simulink library "xps_library"  (R2012b)
settings: Solver=ode45  SolverMode=SingleTasking  StartTime=0.0  StopTime=10.0  RelTol=1e-3
undefined symbols (not defined in the file): sys_clk, xps_library_software_register_user_data_in
libraries: xbsIndex_r4 x788, simulink x100, dspsigops x81, casper_library x62, xps_library x24, casper_library_misc x3, xbsIndex_r3 x2
(part 5 of 9)

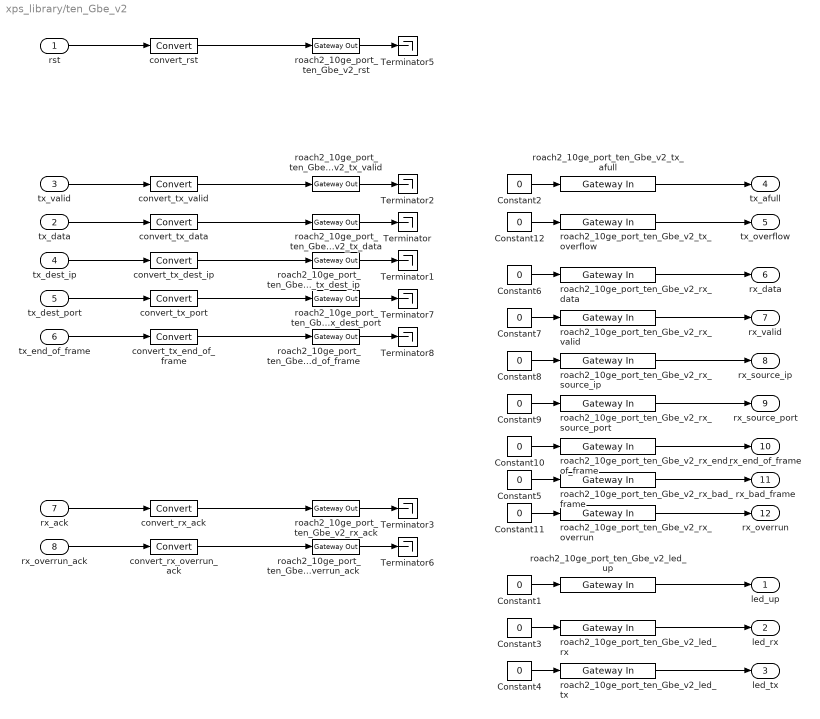
== system xps_library/ten_Gbe_v2 ==
  rst : Inport
  tx_data : Inport  Port=2
  tx_valid : Inport  Port=3
  tx_dest_ip : Inport  Port=4
  tx_dest_port : Inport  Port=5
  tx_end_of_frame : Inport  Port=6
  rx_ack : Inport  Port=7
  rx_overrun_ack : Inport  Port=8
  Constant{1..12} (12 alike) : Constant  Value=0
  Terminator{,1..3,5..8} (8 alike) : Terminator
  convert_rst : xbsIndex_r4/Convert  arith_type=Boolean  n_bits=64  bin_pt=0  quantization=Truncate  overflow=Wrap  latency=0  dbl_ovrd=off  pipeline=off  block_type=convert
      settings: xl_area=[0, 0, 0, 0, 0, 0, 0]
  convert_rx_ack : xbsIndex_r4/Convert  arith_type=Boolean  n_bits=64  bin_pt=0  quantization=Truncate  overflow=Wrap  latency=0  dbl_ovrd=off  pipeline=off  block_type=convert
      settings: xl_area=[0, 0, 0, 0, 0, 0, 0]
  convert_rx_overrun_ack : xbsIndex_r4/Convert  arith_type=Boolean  n_bits=64  bin_pt=0  quantization=Truncate  overflow=Wrap  latency=0  dbl_ovrd=off  pipeline=off  block_type=convert
      settings: xl_area=[0, 0, 0, 0, 0, 0, 0]
  convert_tx_data : xbsIndex_r4/Convert  arith_type=Unsigned  n_bits=64  bin_pt=0  quantization=Truncate  overflow=Wrap  latency=0  dbl_ovrd=off  pipeline=off  block_type=convert
      settings: xl_area=[0, 0, 0, 0, 0, 0, 0]
  convert_tx_dest_ip : xbsIndex_r4/Convert  arith_type=Unsigned  n_bits=32  bin_pt=0  quantization=Truncate  overflow=Wrap  latency=0  dbl_ovrd=off  pipeline=off  block_type=convert
      settings: xl_area=[0, 0, 0, 0, 0, 0, 0]
  convert_tx_end_of_frame : xbsIndex_r4/Convert  arith_type=Boolean  n_bits=1  bin_pt=0  quantization=Truncate  overflow=Wrap  latency=0  dbl_ovrd=off  pipeline=off  block_type=convert
      settings: xl_area=[0, 0, 0, 0, 0, 0, 0]
  convert_tx_port : xbsIndex_r4/Convert  arith_type=Unsigned  n_bits=16  bin_pt=0  quantization=Truncate  overflow=Wrap  latency=0  dbl_ovrd=off  pipeline=off  block_type=convert
      settings: xl_area=[0, 0, 0, 0, 0, 0, 0]
  convert_tx_valid : xbsIndex_r4/Convert  arith_type=Boolean  n_bits=1  bin_pt=0  quantization=Truncate  overflow=Wrap  latency=0  dbl_ovrd=off  pipeline=off  block_type=convert
      settings: xl_area=[0, 0, 0, 0, 0, 0, 0]
  roach2_10ge_port_ten_Gbe_v2_led_rx : xbsIndex_r4/Gateway In  arith_type=Boolean  n_bits=1  bin_pt=0  quantization=Truncate  overflow=Wrap  period=1  dbl_ovrd=off  timing_constraint=None  locs_specified=off  LOCs={}  hdl_port=on  block_type=gatewayin
      settings: infoedit="Gateway in block.  Converts inputs of type Simulink integer, double and fixed point to  Xilinx fixed point type.<P><P>Hardware notes:  In hardware these blocks become top level input ports."  xl_area=[0, 0, 0, 0, 0, 0, 0]
  roach2_10ge_port_ten_Gbe_v2_led_tx : xbsIndex_r4/Gateway In  arith_type=Boolean  n_bits=1  bin_pt=0  quantization=Truncate  overflow=Wrap  period=1  dbl_ovrd=off  timing_constraint=None  locs_specified=off  LOCs={}  hdl_port=on  block_type=gatewayin
      settings: infoedit="Gateway in block.  Converts inputs of type Simulink integer, double and fixed point to  Xilinx fixed point type.<P><P>Hardware notes:  In hardware these blocks become top level input ports."  xl_area=[0, 0, 0, 0, 0, 0, 0]
  roach2_10ge_port_ten_Gbe_v2_led_up : xbsIndex_r4/Gateway In  arith_type=Boolean  n_bits=1  bin_pt=0  quantization=Truncate  overflow=Wrap  period=1  dbl_ovrd=off  timing_constraint=None  locs_specified=off  LOCs={}  hdl_port=on  block_type=gatewayin
      settings: infoedit="Gateway in block.  Converts inputs of type Simulink integer, double and fixed point to  Xilinx fixed point type.<P><P>Hardware notes:  In hardware these blocks become top level input ports."  xl_area=[0, 0, 0, 0, 0, 0, 0]
  roach2_10ge_port_ten_Gbe_v2_rst : xbsIndex_r4/Gateway Out  hdl_port=on  timing_constraint=None  locs_specified=off  LOCs={}  block_type=gatewayout
      settings: infoedit="Gateway out block.  Converts Xilinx fixed point inputs into ouputs of type Simulink integer, double, or fixed point.<P><P>Hardware notes:  In hardware these blocks become top level output ports or are discarded, depending on how they are configured."  xl_area=[0, 0, 0, 0, 0, 0, 0]
  roach2_10ge_port_ten_Gbe_v2_rx_ack : xbsIndex_r4/Gateway Out  hdl_port=on  timing_constraint=None  locs_specified=off  LOCs={}  block_type=gatewayout
      settings: infoedit="Gateway out block.  Converts Xilinx fixed point inputs into ouputs of type Simulink integer, double, or fixed point.<P><P>Hardware notes:  In hardware these blocks become top level output ports or are discarded, depending on how they are configured."  xl_area=[0, 0, 0, 0, 0, 0, 0]
  roach2_10ge_port_ten_Gbe_v2_rx_bad_frame : xbsIndex_r4/Gateway In  arith_type=Boolean  n_bits=1  bin_pt=0  quantization=Truncate  overflow=Wrap  period=1  dbl_ovrd=off  timing_constraint=None  locs_specified=off  LOCs={}  hdl_port=on  block_type=gatewayin
      settings: infoedit="Gateway in block.  Converts inputs of type Simulink integer, double and fixed point to  Xilinx fixed point type.<P><P>Hardware notes:  In hardware these blocks become top level input ports."  xl_area=[0, 0, 0, 0, 0, 0, 0]
  roach2_10ge_port_ten_Gbe_v2_rx_data : xbsIndex_r4/Gateway In  arith_type=Unsigned  n_bits=64  bin_pt=0  quantization=Truncate  overflow=Wrap  period=1  dbl_ovrd=off  timing_constraint=None  locs_specified=off  LOCs={}  hdl_port=on  block_type=gatewayin
      settings: infoedit="Gateway in block.  Converts inputs of type Simulink integer, double and fixed point to  Xilinx fixed point type.<P><P>Hardware notes:  In hardware these blocks become top level input ports."  xl_area=[0, 0, 0, 0, 0, 0, 0]
  roach2_10ge_port_ten_Gbe_v2_rx_end_of_frame : xbsIndex_r4/Gateway In  arith_type=Boolean  n_bits=1  bin_pt=0  quantization=Truncate  overflow=Wrap  period=1  dbl_ovrd=off  timing_constraint=None  locs_specified=off  LOCs={}  hdl_port=on  block_type=gatewayin
      settings: infoedit="Gateway in block.  Converts inputs of type Simulink integer, double and fixed point to  Xilinx fixed point type.<P><P>Hardware notes:  In hardware these blocks become top level input ports."  xl_area=[0, 0, 0, 0, 0, 0, 0]
  roach2_10ge_port_ten_Gbe_v2_rx_overrun : xbsIndex_r4/Gateway In  arith_type=Boolean  n_bits=1  bin_pt=0  quantization=Truncate  overflow=Wrap  period=1  dbl_ovrd=off  timing_constraint=None  locs_specified=off  LOCs={}  hdl_port=on  block_type=gatewayin
      settings: infoedit="Gateway in block.  Converts inputs of type Simulink integer, double and fixed point to  Xilinx fixed point type.<P><P>Hardware notes:  In hardware these blocks become top level input ports."  xl_area=[0, 0, 0, 0, 0, 0, 0]
  roach2_10ge_port_ten_Gbe_v2_rx_overrun_ack : xbsIndex_r4/Gateway Out  hdl_port=on  timing_constraint=None  locs_specified=off  LOCs={}  block_type=gatewayout
      settings: infoedit="Gateway out block.  Converts Xilinx fixed point inputs into ouputs of type Simulink integer, double, or fixed point.<P><P>Hardware notes:  In hardware these blocks become top level output ports or are discarded, depending on how they are configured."  xl_area=[0, 0, 0, 0, 0, 0, 0]
  roach2_10ge_port_ten_Gbe_v2_rx_source_ip : xbsIndex_r4/Gateway In  arith_type=Unsigned  n_bits=32  bin_pt=0  quantization=Truncate  overflow=Wrap  period=1  dbl_ovrd=off  timing_constraint=None  locs_specified=off  LOCs={}  hdl_port=on  block_type=gatewayin
      settings: infoedit="Gateway in block.  Converts inputs of type Simulink integer, double and fixed point to  Xilinx fixed point type.<P><P>Hardware notes:  In hardware these blocks become top level input ports."  xl_area=[0, 0, 0, 0, 0, 0, 0]
  roach2_10ge_port_ten_Gbe_v2_rx_source_port : xbsIndex_r4/Gateway In  arith_type=Unsigned  n_bits=16  bin_pt=0  quantization=Truncate  overflow=Wrap  period=1  dbl_ovrd=off  timing_constraint=None  locs_specified=off  LOCs={}  hdl_port=on  block_type=gatewayin
      settings: infoedit="Gateway in block.  Converts inputs of type Simulink integer, double and fixed point to  Xilinx fixed point type.<P><P>Hardware notes:  In hardware these blocks become top level input ports."  xl_area=[0, 0, 0, 0, 0, 0, 0]
  roach2_10ge_port_ten_Gbe_v2_rx_valid : xbsIndex_r4/Gateway In  arith_type=Boolean  n_bits=1  bin_pt=0  quantization=Truncate  overflow=Wrap  period=1  dbl_ovrd=off  timing_constraint=None  locs_specified=off  LOCs={}  hdl_port=on  block_type=gatewayin
      settings: infoedit="Gateway in block.  Converts inputs of type Simulink integer, double and fixed point to  Xilinx fixed point type.<P><P>Hardware notes:  In hardware these blocks become top level input ports."  xl_area=[0, 0, 0, 0, 0, 0, 0]
  roach2_10ge_port_ten_Gbe_v2_tx_afull : xbsIndex_r4/Gateway In  arith_type=Boolean  n_bits=1  bin_pt=0  quantization=Truncate  overflow=Wrap  period=1  dbl_ovrd=off  timing_constraint=None  locs_specified=off  LOCs={}  hdl_port=on  block_type=gatewayin
      settings: infoedit="Gateway in block.  Converts inputs of type Simulink integer, double and fixed point to  Xilinx fixed point type.<P><P>Hardware notes:  In hardware these blocks become top level input ports."  xl_area=[0, 0, 0, 0, 0, 0, 0]
  roach2_10ge_port_ten_Gbe_v2_tx_data : xbsIndex_r4/Gateway Out  hdl_port=on  timing_constraint=None  locs_specified=off  LOCs={}  block_type=gatewayout
      settings: infoedit="Gateway out block.  Converts Xilinx fixed point inputs into ouputs of type Simulink integer, double, or fixed point.<P><P>Hardware notes:  In hardware these blocks become top level output ports or are discarded, depending on how they are configured."  xl_area=[0, 0, 0, 0, 0, 0, 0]
  roach2_10ge_port_ten_Gbe_v2_tx_dest_ip : xbsIndex_r4/Gateway Out  hdl_port=on  timing_constraint=None  locs_specified=off  LOCs={}  block_type=gatewayout
      settings: infoedit="Gateway out block.  Converts Xilinx fixed point inputs into ouputs of type Simulink integer, double, or fixed point.<P><P>Hardware notes:  In hardware these blocks become top level output ports or are discarded, depending on how they are configured."  xl_area=[0, 0, 0, 0, 0, 0, 0]
  roach2_10ge_port_ten_Gbe_v2_tx_dest_port : xbsIndex_r4/Gateway Out  hdl_port=on  timing_constraint=None  locs_specified=off  LOCs={}  block_type=gatewayout
      settings: infoedit="Gateway out block.  Converts Xilinx fixed point inputs into ouputs of type Simulink integer, double, or fixed point.<P><P>Hardware notes:  In hardware these blocks become top level output ports or are discarded, depending on how they are configured."  xl_area=[0, 0, 0, 0, 0, 0, 0]
  roach2_10ge_port_ten_Gbe_v2_tx_end_of_frame : xbsIndex_r4/Gateway Out  hdl_port=on  timing_constraint=None  locs_specified=off  LOCs={}  block_type=gatewayout
      settings: infoedit="Gateway out block.  Converts Xilinx fixed point inputs into ouputs of type Simulink integer, double, or fixed point.<P><P>Hardware notes:  In hardware these blocks become top level output ports or are discarded, depending on how they are configured."  xl_area=[0, 0, 0, 0, 0, 0, 0]
  roach2_10ge_port_ten_Gbe_v2_tx_overflow : xbsIndex_r4/Gateway In  arith_type=Boolean  n_bits=1  bin_pt=0  quantization=Truncate  overflow=Wrap  period=1  dbl_ovrd=off  timing_constraint=None  locs_specified=off  LOCs={}  hdl_port=on  block_type=gatewayin
      settings: infoedit="Gateway in block.  Converts inputs of type Simulink integer, double and fixed point to  Xilinx fixed point type.<P><P>Hardware notes:  In hardware these blocks become top level input ports."  xl_area=[0, 0, 0, 0, 0, 0, 0]
  roach2_10ge_port_ten_Gbe_v2_tx_valid : xbsIndex_r4/Gateway Out  hdl_port=on  timing_constraint=None  locs_specified=off  LOCs={}  block_type=gatewayout
      settings: infoedit="Gateway out block.  Converts Xilinx fixed point inputs into ouputs of type Simulink integer, double, or fixed point.<P><P>Hardware notes:  In hardware these blocks become top level output ports or are discarded, depending on how they are configured."  xl_area=[0, 0, 0, 0, 0, 0, 0]
  led_up : Outport
  led_rx : Outport  Port=2
  led_tx : Outport  Port=3
  tx_afull : Outport  Port=4
  tx_overflow : Outport  Port=5
  rx_data : Outport  Port=6
  rx_valid : Outport  Port=7
  rx_source_ip : Outport  Port=8
  rx_source_port : Outport  Port=9
  rx_end_of_frame : Outport  Port=10
  rx_bad_frame : Outport  Port=11
  rx_overrun : Outport  Port=12
  wires:
  roach2_10ge_port_ten_Gbe_v2_led_tx/1 -> led_tx/1
  Constant4/1 -> roach2_10ge_port_ten_Gbe_v2_led_tx/1
  roach2_10ge_port_ten_Gbe_v2_led_rx/1 -> led_rx/1
  Constant3/1 -> roach2_10ge_port_ten_Gbe_v2_led_rx/1
  roach2_10ge_port_ten_Gbe_v2_led_up/1 -> led_up/1
  Constant1/1 -> roach2_10ge_port_ten_Gbe_v2_led_up/1
  roach2_10ge_port_ten_Gbe_v2_rx_end_of_frame/1 -> rx_end_of_frame/1
  Constant10/1 -> roach2_10ge_port_ten_Gbe_v2_rx_end_of_frame/1
  roach2_10ge_port_ten_Gbe_v2_rx_source_port/1 -> rx_source_port/1
  Constant9/1 -> roach2_10ge_port_ten_Gbe_v2_rx_source_port/1
  Constant8/1 -> roach2_10ge_port_ten_Gbe_v2_rx_source_ip/1
  roach2_10ge_port_ten_Gbe_v2_rx_source_ip/1 -> rx_source_ip/1
  roach2_10ge_port_ten_Gbe_v2_tx_end_of_frame/1 -> Terminator8/1
  convert_tx_end_of_frame/1 -> roach2_10ge_port_ten_Gbe_v2_tx_end_of_frame/1
  tx_end_of_frame/1 -> convert_tx_end_of_frame/1
  roach2_10ge_port_ten_Gbe_v2_tx_dest_port/1 -> Terminator7/1
  convert_tx_port/1 -> roach2_10ge_port_ten_Gbe_v2_tx_dest_port/1
  tx_dest_port/1 -> convert_tx_port/1
  roach2_10ge_port_ten_Gbe_v2_rst/1 -> Terminator5/1
  convert_rst/1 -> roach2_10ge_port_ten_Gbe_v2_rst/1
  rst/1 -> convert_rst/1
  roach2_10ge_port_ten_Gbe_v2_rx_valid/1 -> rx_valid/1
  Constant7/1 -> roach2_10ge_port_ten_Gbe_v2_rx_valid/1
  roach2_10ge_port_ten_Gbe_v2_rx_ack/1 -> Terminator3/1
  Constant6/1 -> roach2_10ge_port_ten_Gbe_v2_rx_data/1
  Constant2/1 -> roach2_10ge_port_ten_Gbe_v2_tx_afull/1
  roach2_10ge_port_ten_Gbe_v2_tx_valid/1 -> Terminator2/1
  roach2_10ge_port_ten_Gbe_v2_tx_dest_ip/1 -> Terminator1/1
  roach2_10ge_port_ten_Gbe_v2_tx_data/1 -> Terminator/1
  roach2_10ge_port_ten_Gbe_v2_tx_afull/1 -> tx_afull/1
  convert_tx_valid/1 -> roach2_10ge_port_ten_Gbe_v2_tx_valid/1
  tx_valid/1 -> convert_tx_valid/1
  convert_tx_dest_ip/1 -> roach2_10ge_port_ten_Gbe_v2_tx_dest_ip/1
  tx_dest_ip/1 -> convert_tx_dest_ip/1
  convert_tx_data/1 -> roach2_10ge_port_ten_Gbe_v2_tx_data/1
  tx_data/1 -> convert_tx_data/1
  roach2_10ge_port_ten_Gbe_v2_rx_data/1 -> rx_data/1
  convert_rx_ack/1 -> roach2_10ge_port_ten_Gbe_v2_rx_ack/1
  rx_ack/1 -> convert_rx_ack/1
  roach2_10ge_port_ten_Gbe_v2_rx_bad_frame/1 -> rx_bad_frame/1
  Constant5/1 -> roach2_10ge_port_ten_Gbe_v2_rx_bad_frame/1
  roach2_10ge_port_ten_Gbe_v2_rx_overrun/1 -> rx_overrun/1
  Constant11/1 -> roach2_10ge_port_ten_Gbe_v2_rx_overrun/1
  roach2_10ge_port_ten_Gbe_v2_rx_overrun_ack/1 -> Terminator6/1
  convert_rx_overrun_ack/1 -> roach2_10ge_port_ten_Gbe_v2_rx_overrun_ack/1
  rx_overrun_ack/1 -> convert_rx_overrun_ack/1
  Constant12/1 -> roach2_10ge_port_ten_Gbe_v2_tx_overflow/1
  roach2_10ge_port_ten_Gbe_v2_tx_overflow/1 -> tx_overflow/1

== system xps_library/ADCs/adc083000_ctrl ==
  conf : Inport
  sdata_bus : Inport  Port=2
  Convert : xbsIndex_r4/Convert  arith_type=Unsigned  n_bits=3  bin_pt=0  quantization=Truncate  overflow=Wrap  latency=2  dbl_ovrd=off  pipeline=off  block_type=convert
      settings: block_version=11.4
  Convert1 : xbsIndex_r4/Convert  arith_type=Unsigned  n_bits=32  bin_pt=0  quantization=Truncate  overflow=Wrap  latency=2  dbl_ovrd=off  pipeline=off  block_type=convert
      settings: block_version=11.4
  Slice : xbsIndex_r4/Slice  nbits=3  boolean_output=off  mode=Lower Bit Location + Width  bit1=0  base1=MSB of Input  bit0=0  base0=LSB of Input  dbl_ovrd=off  block_type=slice
  Terminator : Terminator
  Terminator1 : Terminator
  xps_library_ADCs_adc083000_ctrl_conf : xbsIndex_r4/Gateway Out  hdl_port=on  timing_constraint=None  locs_specified=off  LOCs={}  block_type=gatewayout
      settings: infoedit="Gateway out block.  Converts Xilinx fixed point inputs into ouputs of type Simulink integer, double, or fixed point.<br><br>Hardware notes:  In hardware these blocks become top level output ports or are discarded, depending on how they are configured."  block_version=11.4
  xps_library_ADCs_adc083000_ctrl_sdata_bus : xbsIndex_r4/Gateway Out  hdl_port=on  timing_constraint=None  locs_specified=off  LOCs={}  block_type=gatewayout
      settings: infoedit="Gateway out block.  Converts Xilinx fixed point inputs into ouputs of type Simulink integer, double, or fixed point.<br><br>Hardware notes:  In hardware these blocks become top level output ports or are discarded, depending on how they are configured."  block_version=11.4
  wires:
  xps_library_ADCs_adc083000_ctrl_sdata_bus/1 -> Terminator1/1
  xps_library_ADCs_adc083000_ctrl_conf/1 -> Terminator/1
  Convert1/1 -> xps_library_ADCs_adc083000_ctrl_sdata_bus/1
  Slice/1 -> Convert/1
  conf/1 -> Slice/1
  Convert/1 -> xps_library_ADCs_adc083000_ctrl_conf/1
  sdata_bus/1 -> Convert1/1

== system xps_library/ADCs/adc2x14_400 ==
  adc_snap_test_zdock0_adc2x14_400_user_data_i0 : xbsIndex_r4/Gateway In  arith_type=Unsigned  n_bits=14  bin_pt=0  quantization=Truncate  overflow=Wrap  period=1  dbl_ovrd=off  timing_constraint=None  locs_specified=off  LOCs={}  hdl_port=on  block_type=gatewayin
      settings: infoedit="Gateway in block.  Converts inputs of type Simulink integer, double and fixed point to  Xilinx fixed point type.<P><P>Hardware notes:  In hardware these blocks become top level input ports."  xl_area=[0, 0, 0, 0, 0, 0, 0]  block_version=10.1.3
  adc_snap_test_zdock0_adc2x14_400_user_data_i1 : xbsIndex_r4/Gateway In  arith_type=Unsigned  n_bits=14  bin_pt=0  quantization=Truncate  overflow=Wrap  period=1  dbl_ovrd=off  timing_constraint=None  locs_specified=off  LOCs={}  hdl_port=on  block_type=gatewayin
      settings: infoedit="Gateway in block.  Converts inputs of type Simulink integer, double and fixed point to  Xilinx fixed point type.<P><P>Hardware notes:  In hardware these blocks become top level input ports."  xl_area=[0, 0, 0, 0, 0, 0, 0]  block_version=10.1.3
  adc_snap_test_zdock0_adc2x14_400_user_data_q0 : xbsIndex_r4/Gateway In  arith_type=Unsigned  n_bits=14  bin_pt=0  quantization=Truncate  overflow=Wrap  period=1  dbl_ovrd=off  timing_constraint=None  locs_specified=off  LOCs={}  hdl_port=on  block_type=gatewayin
      settings: infoedit="Gateway in block.  Converts inputs of type Simulink integer, double and fixed point to  Xilinx fixed point type.<P><P>Hardware notes:  In hardware these blocks become top level input ports."  xl_area=[0, 0, 0, 0, 0, 0, 0]  block_version=10.1.3
  adc_snap_test_zdock0_adc2x14_400_user_data_q1 : xbsIndex_r4/Gateway In  arith_type=Unsigned  n_bits=14  bin_pt=0  quantization=Truncate  overflow=Wrap  period=1  dbl_ovrd=off  timing_constraint=None  locs_specified=off  LOCs={}  hdl_port=on  block_type=gatewayin
      settings: infoedit="Gateway in block.  Converts inputs of type Simulink integer, double and fixed point to  Xilinx fixed point type.<P><P>Hardware notes:  In hardware these blocks become top level input ports."  xl_area=[0, 0, 0, 0, 0, 0, 0]  block_version=10.1.3
  adc_snap_test_zdock0_adc2x14_400_user_sync : xbsIndex_r4/Gateway In  arith_type=Boolean  n_bits=1  bin_pt=0  quantization=Truncate  overflow=Wrap  period=1  dbl_ovrd=off  timing_constraint=None  locs_specified=off  LOCs={}  hdl_port=on  block_type=gatewayin
      settings: infoedit="Gateway in block.  Converts inputs of type Simulink integer, double and fixed point to  Xilinx fixed point type.<P><P>Hardware notes:  In hardware these blocks become top level input ports."  xl_area=[0, 0, 0, 0, 0, 0, 0]  block_version=10.1.3
  conv : Subsystem
      mask help:
      | Converts an (12-bit) unsigned number to 2's complement.
      | This block should eventually be able to handle arbitrary
      | width inputs.
  conv1 : Subsystem
      mask help:
      | Converts an (12-bit) unsigned number to 2's complement.
      | This block should eventually be able to handle arbitrary
      | width inputs.
  conv2 : Subsystem
      mask help:
      | Converts an (12-bit) unsigned number to 2's complement.
      | This block should eventually be able to handle arbitrary
      | width inputs.
  conv3 : Subsystem
      mask help:
      | Converts an (12-bit) unsigned number to 2's complement.
      | This block should eventually be able to handle arbitrary
      | width inputs.
  data_i0 : Outport
  data_i1 : Outport  Port=2
  data_q0 : Outport  Port=3
  data_q1 : Outport  Port=4
  sync : Outport  Port=5
  wires:
  adc_snap_test_zdock0_adc2x14_400_user_sync/1 -> sync/1
  adc_snap_test_zdock0_adc2x14_400_user_data_i0/1 -> conv/1(In1)
  conv/1(Out1) -> data_i0/1
  adc_snap_test_zdock0_adc2x14_400_user_data_q0/1 -> conv2/1(In1)
  conv2/1(Out1) -> data_q0/1
  adc_snap_test_zdock0_adc2x14_400_user_data_i1/1 -> conv1/1(In1)
  conv1/1(Out1) -> data_i1/1
  adc_snap_test_zdock0_adc2x14_400_user_data_q1/1 -> conv3/1(In1)
  conv3/1(Out1) -> data_q1/1

== system xps_library/ADCs/adc2x14_400_4x ==
  conv : Subsystem
      mask help:
      | Converts an (14-bit) unsigned number to 2's complement.
      | This block should eventually be able to handle arbitrary
      | width inputs.
  conv1 : Subsystem
      mask help:
      | Converts an (14-bit) unsigned number to 2's complement.
      | This block should eventually be able to handle arbitrary
      | width inputs.
  conv2 : Subsystem
      mask help:
      | Converts an (14-bit) unsigned number to 2's complement.
      | This block should eventually be able to handle arbitrary
      | width inputs.
  conv3 : Subsystem
      mask help:
      | Converts an (14-bit) unsigned number to 2's complement.
      | This block should eventually be able to handle arbitrary
      | width inputs.
  conv4 : Subsystem
      mask help:
      | Converts an (14-bit) unsigned number to 2's complement.
      | This block should eventually be able to handle arbitrary
      | width inputs.
  conv5 : Subsystem
      mask help:
      | Converts an (14-bit) unsigned number to 2's complement.
      | This block should eventually be able to handle arbitrary
      | width inputs.
  conv6 : Subsystem
      mask help:
      | Converts an (14-bit) unsigned number to 2's complement.
      | This block should eventually be able to handle arbitrary
      | width inputs.
  conv7 : Subsystem
      mask help:
      | Converts an (14-bit) unsigned number to 2's complement.
      | This block should eventually be able to handle arbitrary
      | width inputs.
  xps_library_ADCs_adc2x14_400_4x_user_data_i{0..3} (4 alike) : xbsIndex_r4/Gateway In  arith_type=Unsigned  n_bits=14  bin_pt=0  quantization=Truncate  overflow=Wrap  period=1  dbl_ovrd=off  timing_constraint=None  locs_specified=off  LOCs={}  block_type=gatewayin
      settings: infoedit="Gateway in block.  Converts inputs of type Simulink integer, double and fixed point to  Xilinx fixed point type.<P><P>Hardware notes:  In hardware these blocks become top level input ports."  xl_area=[0, 0, 0, 0, 0, 0, 0]  block_version=10.1.3
  xps_library_ADCs_adc2x14_400_4x_user_data_q{0..3} (4 alike) : xbsIndex_r4/Gateway In  arith_type=Unsigned  n_bits=14  bin_pt=0  quantization=Truncate  overflow=Wrap  period=1  dbl_ovrd=off  timing_constraint=None  locs_specified=off  LOCs={}  block_type=gatewayin
      settings: infoedit="Gateway in block.  Converts inputs of type Simulink integer, double and fixed point to  Xilinx fixed point type.<P><P>Hardware notes:  In hardware these blocks become top level input ports."  xl_area=[0, 0, 0, 0, 0, 0, 0]  block_version=10.1.3
  xps_library_ADCs_adc2x14_400_4x_user_sync : xbsIndex_r4/Gateway In  arith_type=Boolean  n_bits=1  bin_pt=0  quantization=Truncate  overflow=Wrap  period=1  dbl_ovrd=off  timing_constraint=None  locs_specified=off  LOCs={}  block_type=gatewayin
      settings: infoedit="Gateway in block.  Converts inputs of type Simulink integer, double and fixed point to  Xilinx fixed point type.<P><P>Hardware notes:  In hardware these blocks become top level input ports."  xl_area=[0, 0, 0, 0, 0, 0, 0]  block_version=10.1.3
  data_i0 : Outport
  data_i1 : Outport  Port=2
  data_i2 : Outport  Port=3
  data_i3 : Outport  Port=4
  data_q0 : Outport  Port=5
  data_q1 : Outport  Port=6
  data_q2 : Outport  Port=7
  data_q3 : Outport  Port=8
  sync : Outport  Port=9
  wires:
  conv5/1(Out1) -> data_q1/1
  xps_library_ADCs_adc2x14_400_4x_user_data_q1/1 -> conv5/1(In1)
  conv1/1(Out1) -> data_i1/1
  xps_library_ADCs_adc2x14_400_4x_user_data_i1/1 -> conv1/1(In1)
  conv4/1(Out1) -> data_q0/1
  xps_library_ADCs_adc2x14_400_4x_user_data_q0/1 -> conv4/1(In1)
  conv/1(Out1) -> data_i0/1
  xps_library_ADCs_adc2x14_400_4x_user_data_i0/1 -> conv/1(In1)
  xps_library_ADCs_adc2x14_400_4x_user_sync/1 -> sync/1
  conv2/1(Out1) -> data_i2/1
  xps_library_ADCs_adc2x14_400_4x_user_data_i2/1 -> conv2/1(In1)
  conv3/1(Out1) -> data_i3/1
  xps_library_ADCs_adc2x14_400_4x_user_data_i3/1 -> conv3/1(In1)
  conv6/1(Out1) -> data_q2/1
  xps_library_ADCs_adc2x14_400_4x_user_data_q2/1 -> conv6/1(In1)
  conv7/1(Out1) -> data_q3/1
  xps_library_ADCs_adc2x14_400_4x_user_data_q3/1 -> conv7/1(In1)

== system xps_library/ADCs/adc_mkid ==
  conv : Subsystem
      mask help:
      | Converts an (12-bit) unsigned number to 2's complement.
      | This block should eventually be able to handle arbitrary
      | width inputs.
  conv1 : Subsystem
      mask help:
      | Converts an (12-bit) unsigned number to 2's complement.
      | This block should eventually be able to handle arbitrary
      | width inputs.
  conv2 : Subsystem
      mask help:
      | Converts an (12-bit) unsigned number to 2's complement.
      | This block should eventually be able to handle arbitrary
      | width inputs.
  conv3 : Subsystem
      mask help:
      | Converts an (12-bit) unsigned number to 2's complement.
      | This block should eventually be able to handle arbitrary
      | width inputs.
  xps_library_ADCs_adc_mkid_user_data_i0 : xbsIndex_r4/Gateway In  arith_type=Unsigned  n_bits=12  bin_pt=0  quantization=Truncate  overflow=Wrap  period=1  dbl_ovrd=off  timing_constraint=None  locs_specified=off  LOCs={}  hdl_port=on  block_type=gatewayin
      settings: infoedit="Gateway in block.  Converts inputs of type Simulink integer, double and fixed point to  Xilinx fixed point type.<P><P>Hardware notes:  In hardware these blocks become top level input ports."  xl_area=[0, 0, 0, 0, 0, 0, 0]  block_version=10.1.3
  xps_library_ADCs_adc_mkid_user_data_i1 : xbsIndex_r4/Gateway In  arith_type=Unsigned  n_bits=12  bin_pt=0  quantization=Truncate  overflow=Wrap  period=1  dbl_ovrd=off  timing_constraint=None  locs_specified=off  LOCs={}  hdl_port=on  block_type=gatewayin
      settings: infoedit="Gateway in block.  Converts inputs of type Simulink integer, double and fixed point to  Xilinx fixed point type.<P><P>Hardware notes:  In hardware these blocks become top level input ports."  xl_area=[0, 0, 0, 0, 0, 0, 0]  block_version=10.1.3
  xps_library_ADCs_adc_mkid_user_data_q0 : xbsIndex_r4/Gateway In  arith_type=Unsigned  n_bits=12  bin_pt=0  quantization=Truncate  overflow=Wrap  period=1  dbl_ovrd=off  timing_constraint=None  locs_specified=off  LOCs={}  hdl_port=on  block_type=gatewayin
      settings: infoedit="Gateway in block.  Converts inputs of type Simulink integer, double and fixed point to  Xilinx fixed point type.<P><P>Hardware notes:  In hardware these blocks become top level input ports."  xl_area=[0, 0, 0, 0, 0, 0, 0]  block_version=10.1.3
  xps_library_ADCs_adc_mkid_user_data_q1 : xbsIndex_r4/Gateway In  arith_type=Unsigned  n_bits=12  bin_pt=0  quantization=Truncate  overflow=Wrap  period=1  dbl_ovrd=off  timing_constraint=None  locs_specified=off  LOCs={}  hdl_port=on  block_type=gatewayin
      settings: infoedit="Gateway in block.  Converts inputs of type Simulink integer, double and fixed point to  Xilinx fixed point type.<P><P>Hardware notes:  In hardware these blocks become top level input ports."  xl_area=[0, 0, 0, 0, 0, 0, 0]  block_version=10.1.3
  xps_library_ADCs_adc_mkid_user_sync : xbsIndex_r4/Gateway In  arith_type=Boolean  n_bits=1  bin_pt=0  quantization=Truncate  overflow=Wrap  period=1  dbl_ovrd=off  timing_constraint=None  locs_specified=off  LOCs={}  hdl_port=on  block_type=gatewayin
      settings: infoedit="Gateway in block.  Converts inputs of type Simulink integer, double and fixed point to  Xilinx fixed point type.<P><P>Hardware notes:  In hardware these blocks become top level input ports."  xl_area=[0, 0, 0, 0, 0, 0, 0]  block_version=10.1.3
  data_i0 : Outport
  data_i1 : Outport  Port=2
  data_q0 : Outport  Port=3
  data_q1 : Outport  Port=4
  sync : Outport  Port=5
  wires:
  xps_library_ADCs_adc_mkid_user_sync/1 -> sync/1
  xps_library_ADCs_adc_mkid_user_data_i0/1 -> conv/1(In1)
  conv/1(Out1) -> data_i0/1
  xps_library_ADCs_adc_mkid_user_data_q0/1 -> conv2/1(In1)
  conv2/1(Out1) -> data_q0/1
  xps_library_ADCs_adc_mkid_user_data_i1/1 -> conv1/1(In1)
  conv1/1(Out1) -> data_i1/1
  xps_library_ADCs_adc_mkid_user_data_q1/1 -> conv3/1(In1)
  conv3/1(Out1) -> data_q1/1

== system xps_library/ADCs/adc_mkid_4x ==
  conv : Subsystem
      mask help:
      | Converts an (12-bit) unsigned number to 2's complement.
      | This block should eventually be able to handle arbitrary
      | width inputs.
  conv1 : Subsystem
      mask help:
      | Converts an (12-bit) unsigned number to 2's complement.
      | This block should eventually be able to handle arbitrary
      | width inputs.
  conv2 : Subsystem
      mask help:
      | Converts an (12-bit) unsigned number to 2's complement.
      | This block should eventually be able to handle arbitrary
      | width inputs.
  conv3 : Subsystem
      mask help:
      | Converts an (12-bit) unsigned number to 2's complement.
      | This block should eventually be able to handle arbitrary
      | width inputs.
  conv4 : Subsystem
      mask help:
      | Converts an (12-bit) unsigned number to 2's complement.
      | This block should eventually be able to handle arbitrary
      | width inputs.
  conv5 : Subsystem
      mask help:
      | Converts an (12-bit) unsigned number to 2's complement.
      | This block should eventually be able to handle arbitrary
      | width inputs.
  conv6 : Subsystem
      mask help:
      | Converts an (12-bit) unsigned number to 2's complement.
      | This block should eventually be able to handle arbitrary
      | width inputs.
  conv7 : Subsystem
      mask help:
      | Converts an (12-bit) unsigned number to 2's complement.
      | This block should eventually be able to handle arbitrary
      | width inputs.
  xps_library_ADCs_adc_mkid_4x_user_data_i{0..3} (4 alike) : xbsIndex_r4/Gateway In  arith_type=Unsigned  n_bits=12  bin_pt=0  quantization=Truncate  overflow=Wrap  period=1  dbl_ovrd=off  timing_constraint=None  locs_specified=off  LOCs={}  block_type=gatewayin
      settings: infoedit="Gateway in block.  Converts inputs of type Simulink integer, double and fixed point to  Xilinx fixed point type.<P><P>Hardware notes:  In hardware these blocks become top level input ports."  xl_area=[0, 0, 0, 0, 0, 0, 0]  block_version=10.1.3
  xps_library_ADCs_adc_mkid_4x_user_data_q{0..3} (4 alike) : xbsIndex_r4/Gateway In  arith_type=Unsigned  n_bits=12  bin_pt=0  quantization=Truncate  overflow=Wrap  period=1  dbl_ovrd=off  timing_constraint=None  locs_specified=off  LOCs={}  block_type=gatewayin
      settings: infoedit="Gateway in block.  Converts inputs of type Simulink integer, double and fixed point to  Xilinx fixed point type.<P><P>Hardware notes:  In hardware these blocks become top level input ports."  xl_area=[0, 0, 0, 0, 0, 0, 0]  block_version=10.1.3
  xps_library_ADCs_adc_mkid_4x_user_sync : xbsIndex_r4/Gateway In  arith_type=Boolean  n_bits=1  bin_pt=0  quantization=Truncate  overflow=Wrap  period=1  dbl_ovrd=off  timing_constraint=None  locs_specified=off  LOCs={}  block_type=gatewayin
      settings: infoedit="Gateway in block.  Converts inputs of type Simulink integer, double and fixed point to  Xilinx fixed point type.<P><P>Hardware notes:  In hardware these blocks become top level input ports."  xl_area=[0, 0, 0, 0, 0, 0, 0]  block_version=10.1.3
  data_i0 : Outport
  data_i1 : Outport  Port=2
  data_i2 : Outport  Port=3
  data_i3 : Outport  Port=4
  data_q0 : Outport  Port=5
  data_q1 : Outport  Port=6
  data_q2 : Outport  Port=7
  data_q3 : Outport  Port=8
  sync : Outport  Port=9
  wires:
  xps_library_ADCs_adc_mkid_4x_user_data_q3/1 -> conv7/1(In1)
  conv7/1(Out1) -> data_q3/1
  xps_library_ADCs_adc_mkid_4x_user_data_q2/1 -> conv6/1(In1)
  conv6/1(Out1) -> data_q2/1
  xps_library_ADCs_adc_mkid_4x_user_data_i3/1 -> conv5/1(In1)
  conv5/1(Out1) -> data_i3/1
  xps_library_ADCs_adc_mkid_4x_user_data_i2/1 -> conv4/1(In1)
  conv4/1(Out1) -> data_i2/1
  xps_library_ADCs_adc_mkid_4x_user_sync/1 -> sync/1
  xps_library_ADCs_adc_mkid_4x_user_data_i0/1 -> conv/1(In1)
  conv/1(Out1) -> data_i0/1
  xps_library_ADCs_adc_mkid_4x_user_data_q0/1 -> conv2/1(In1)
  conv2/1(Out1) -> data_q0/1
  xps_library_ADCs_adc_mkid_4x_user_data_i1/1 -> conv1/1(In1)
  conv1/1(Out1) -> data_i1/1
  xps_library_ADCs_adc_mkid_4x_user_data_q1/1 -> conv3/1(In1)
  conv3/1(Out1) -> data_q1/1

== system xps_library/ADCs/adc_sim ==
  sim_adc_data_in : Inport
  adc_bias : Bias  Bias=128  SaturateOnIntegerOverflow=on
  adc_gain : Gain  Gain=128
  overflow_detector : Subsystem  AncestorBlock=casper_library/Misc/of_detect_bus  mask(of_detect_bus){nStreams=8, bit_width=8}
      mask prompts: nStreams "Number of Streams"; bit_width "Bit Width"
      mask init:
      | adc_overflow_detector_init(gcb, ...
      |     'nStreams', nStreams, ...
      |     'bit_width', bit_width);
  sample0_ds : dspsigops/Downsample  N=8  phase=1  ic=0  smode=Allow multirate  fmode=Maintain input frame size
  sample1_ds : dspsigops/Downsample  N=8  phase=2  ic=0  smode=Allow multirate  fmode=Maintain input frame size
  sample2_ds : dspsigops/Downsample  N=8  phase=3  ic=0  smode=Allow multirate  fmode=Maintain input frame size
  sample3_ds : dspsigops/Downsample  N=8  phase=4  ic=0  smode=Allow multirate  fmode=Maintain input frame size
  sample4_ds : dspsigops/Downsample  N=8  phase=5  ic=0  smode=Allow multirate  fmode=Maintain input frame size
  sample5_ds : dspsigops/Downsample  N=8  phase=6  ic=0  smode=Allow multirate  fmode=Maintain input frame size
  sample6_ds : dspsigops/Downsample  N=8  phase=7  ic=0  smode=Allow multirate  fmode=Maintain input frame size
  sample7_ds : dspsigops/Downsample  N=8  phase=0  ic=0  smode=Allow multirate  fmode=Maintain input frame size
  s0 : Outport
  s1 : Outport  Port=2
  s2 : Outport  Port=3
  s3 : Outport  Port=4
  s4 : Outport  Port=5
  s5 : Outport  Port=6
  s6 : Outport  Port=7
  s7 : Outport  Port=8
  of : Outport  Port=9
  wires:
  sim_adc_data_in/1 -> adc_gain/1
  adc_gain/1 -> adc_bias/1

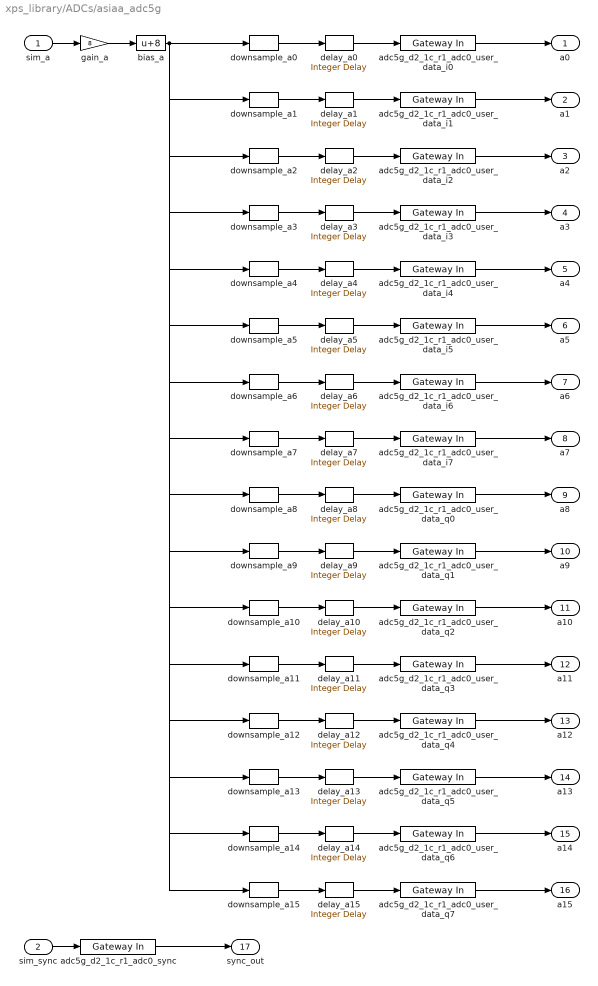
== system xps_library/ADCs/asiaa_adc5g ==
  sim_a : Inport
  sim_sync : Inport  Port=2
  adc5g_d2_1c_r1_adc0_sync : xbsIndex_r4/Gateway In  arith_type=Boolean  n_bits=16  bin_pt=14  quantization="Round  (unbiased: +/- Inf)"  overflow=Saturate  period=1  dbl_ovrd=off  timing_constraint=None  locs_specified=off  LOCs={}  hdl_port=on  block_type=gatewayin
      settings: infoedit="Gateway in block.  Converts inputs of type Simulink integer, double and fixed point to  Xilinx fixed point type.<br><br>Hardware notes:  In hardware these blocks become top level input ports."
  adc5g_d2_1c_r1_adc0_user_data_i{0..7} (8 alike) : xbsIndex_r4/Gateway In  arith_type=Unsigned  n_bits=4  bin_pt=0  quantization=Truncate  overflow=Wrap  period=1  dbl_ovrd=off  timing_constraint=None  locs_specified=off  LOCs={}  hdl_port=on  block_type=gatewayin
      settings: infoedit="Gateway in block.  Converts inputs of type Simulink integer, double and fixed point to  Xilinx fixed point type.<br><br>Hardware notes:  In hardware these blocks become top level input ports."
  adc5g_d2_1c_r1_adc0_user_data_q{0..7} (8 alike) : xbsIndex_r4/Gateway In  arith_type=Unsigned  n_bits=4  bin_pt=0  quantization=Truncate  overflow=Wrap  period=1  dbl_ovrd=off  timing_constraint=None  locs_specified=off  LOCs={}  hdl_port=on  block_type=gatewayin
      settings: infoedit="Gateway in block.  Converts inputs of type Simulink integer, double and fixed point to  Xilinx fixed point type.<br><br>Hardware notes:  In hardware these blocks become top level input ports."
  bias_a : Bias  Bias=8  SaturateOnIntegerOverflow=on
  delay_a0 : simulink/Discrete/Integer Delay  NumDelays=2  InputProcessing=Inherited  vinit=0  samptime=-1
  delay_a{1..15} (15 alike) : simulink/Discrete/Integer Delay  NumDelays=1  InputProcessing=Inherited  vinit=0  samptime=-1
  downsample_a0 : dspsigops/Downsample  N=16  phase=0  InputProcessing=Inherited (this choice will be removed - see release notes)  RateOptions=Enforce single-rate processing  smode=Allow multirate  fmode=Maintain input frame size  ic=0
  downsample_a1 : dspsigops/Downsample  N=16  phase=1  InputProcessing=Inherited (this choice will be removed - see release notes)  RateOptions=Enforce single-rate processing  smode=Allow multirate  fmode=Maintain input frame size  ic=0
  downsample_a10 : dspsigops/Downsample  N=16  phase=10  InputProcessing=Inherited (this choice will be removed - see release notes)  RateOptions=Enforce single-rate processing  smode=Allow multirate  fmode=Maintain input frame size  ic=0
  downsample_a11 : dspsigops/Downsample  N=16  phase=11  InputProcessing=Inherited (this choice will be removed - see release notes)  RateOptions=Enforce single-rate processing  smode=Allow multirate  fmode=Maintain input frame size  ic=0
  downsample_a12 : dspsigops/Downsample  N=16  phase=12  InputProcessing=Inherited (this choice will be removed - see release notes)  RateOptions=Enforce single-rate processing  smode=Allow multirate  fmode=Maintain input frame size  ic=0
  downsample_a13 : dspsigops/Downsample  N=16  phase=13  InputProcessing=Inherited (this choice will be removed - see release notes)  RateOptions=Enforce single-rate processing  smode=Allow multirate  fmode=Maintain input frame size  ic=0
  downsample_a14 : dspsigops/Downsample  N=16  phase=14  InputProcessing=Inherited (this choice will be removed - see release notes)  RateOptions=Enforce single-rate processing  smode=Allow multirate  fmode=Maintain input frame size  ic=0
  downsample_a15 : dspsigops/Downsample  N=16  phase=15  InputProcessing=Inherited (this choice will be removed - see release notes)  RateOptions=Enforce single-rate processing  smode=Allow multirate  fmode=Maintain input frame size  ic=0
  downsample_a2 : dspsigops/Downsample  N=16  phase=2  InputProcessing=Inherited (this choice will be removed - see release notes)  RateOptions=Enforce single-rate processing  smode=Allow multirate  fmode=Maintain input frame size  ic=0
  downsample_a3 : dspsigops/Downsample  N=16  phase=3  InputProcessing=Inherited (this choice will be removed - see release notes)  RateOptions=Enforce single-rate processing  smode=Allow multirate  fmode=Maintain input frame size  ic=0
  downsample_a4 : dspsigops/Downsample  N=16  phase=4  InputProcessing=Inherited (this choice will be removed - see release notes)  RateOptions=Enforce single-rate processing  smode=Allow multirate  fmode=Maintain input frame size  ic=0
  downsample_a5 : dspsigops/Downsample  N=16  phase=5  InputProcessing=Inherited (this choice will be removed - see release notes)  RateOptions=Enforce single-rate processing  smode=Allow multirate  fmode=Maintain input frame size  ic=0
  downsample_a6 : dspsigops/Downsample  N=16  phase=6  InputProcessing=Inherited (this choice will be removed - see release notes)  RateOptions=Enforce single-rate processing  smode=Allow multirate  fmode=Maintain input frame size  ic=0
  downsample_a7 : dspsigops/Downsample  N=16  phase=7  InputProcessing=Inherited (this choice will be removed - see release notes)  RateOptions=Enforce single-rate processing  smode=Allow multirate  fmode=Maintain input frame size  ic=0
  downsample_a8 : dspsigops/Downsample  N=16  phase=8  InputProcessing=Inherited (this choice will be removed - see release notes)  RateOptions=Enforce single-rate processing  smode=Allow multirate  fmode=Maintain input frame size  ic=0
  downsample_a9 : dspsigops/Downsample  N=16  phase=9  InputProcessing=Inherited (this choice will be removed - see release notes)  RateOptions=Enforce single-rate processing  smode=Allow multirate  fmode=Maintain input frame size  ic=0
  gain_a : Gain  Gain=8  SaturateOnIntegerOverflow=on  OutDataTypeStr=Inherit: Same as input  ParamDataTypeStr=Inherit: Same as input
  a0 : Outport
  a1 : Outport  Port=2
  a2 : Outport  Port=3
  a3 : Outport  Port=4
  a4 : Outport  Port=5
  a5 : Outport  Port=6
  a6 : Outport  Port=7
  a7 : Outport  Port=8
  a8 : Outport  Port=9
  a9 : Outport  Port=10
  a10 : Outport  Port=11
  a11 : Outport  Port=12
  a12 : Outport  Port=13
  a13 : Outport  Port=14
  a14 : Outport  Port=15
  a15 : Outport  Port=16
  sync_out : Outport  Port=17
  wires:
  adc5g_d2_1c_r1_adc0_sync/1 -> sync_out/1
  sim_sync/1 -> adc5g_d2_1c_r1_adc0_sync/1
  adc5g_d2_1c_r1_adc0_user_data_q7/1 -> a15/1
  delay_a15/1 -> adc5g_d2_1c_r1_adc0_user_data_q7/1
  downsample_a15/1 -> delay_a15/1
  adc5g_d2_1c_r1_adc0_user_data_q6/1 -> a14/1
  delay_a14/1 -> adc5g_d2_1c_r1_adc0_user_data_q6/1
  downsample_a14/1 -> delay_a14/1
  adc5g_d2_1c_r1_adc0_user_data_q5/1 -> a13/1
  delay_a13/1 -> adc5g_d2_1c_r1_adc0_user_data_q5/1
  downsample_a13/1 -> delay_a13/1
  adc5g_d2_1c_r1_adc0_user_data_q4/1 -> a12/1
  delay_a12/1 -> adc5g_d2_1c_r1_adc0_user_data_q4/1
  downsample_a12/1 -> delay_a12/1
  adc5g_d2_1c_r1_adc0_user_data_q3/1 -> a11/1
  delay_a11/1 -> adc5g_d2_1c_r1_adc0_user_data_q3/1
  downsample_a11/1 -> delay_a11/1
  adc5g_d2_1c_r1_adc0_user_data_q2/1 -> a10/1
  delay_a10/1 -> adc5g_d2_1c_r1_adc0_user_data_q2/1
  downsample_a10/1 -> delay_a10/1
  adc5g_d2_1c_r1_adc0_user_data_q1/1 -> a9/1
  delay_a9/1 -> adc5g_d2_1c_r1_adc0_user_data_q1/1
  downsample_a9/1 -> delay_a9/1
  adc5g_d2_1c_r1_adc0_user_data_q0/1 -> a8/1
  delay_a8/1 -> adc5g_d2_1c_r1_adc0_user_data_q0/1
  downsample_a8/1 -> delay_a8/1
  adc5g_d2_1c_r1_adc0_user_data_i7/1 -> a7/1
  delay_a7/1 -> adc5g_d2_1c_r1_adc0_user_data_i7/1
  downsample_a7/1 -> delay_a7/1
  adc5g_d2_1c_r1_adc0_user_data_i6/1 -> a6/1
  delay_a6/1 -> adc5g_d2_1c_r1_adc0_user_data_i6/1
  downsample_a6/1 -> delay_a6/1
  adc5g_d2_1c_r1_adc0_user_data_i5/1 -> a5/1
  delay_a5/1 -> adc5g_d2_1c_r1_adc0_user_data_i5/1
  downsample_a5/1 -> delay_a5/1
  adc5g_d2_1c_r1_adc0_user_data_i4/1 -> a4/1
  delay_a4/1 -> adc5g_d2_1c_r1_adc0_user_data_i4/1
  downsample_a4/1 -> delay_a4/1
  adc5g_d2_1c_r1_adc0_user_data_i3/1 -> a3/1
  delay_a3/1 -> adc5g_d2_1c_r1_adc0_user_data_i3/1
  downsample_a3/1 -> delay_a3/1
  adc5g_d2_1c_r1_adc0_user_data_i2/1 -> a2/1
  delay_a2/1 -> adc5g_d2_1c_r1_adc0_user_data_i2/1
  downsample_a2/1 -> delay_a2/1
  adc5g_d2_1c_r1_adc0_user_data_i1/1 -> a1/1
  delay_a1/1 -> adc5g_d2_1c_r1_adc0_user_data_i1/1
  downsample_a1/1 -> delay_a1/1
  adc5g_d2_1c_r1_adc0_user_data_i0/1 -> a0/1
  delay_a0/1 -> adc5g_d2_1c_r1_adc0_user_data_i0/1
  downsample_a0/1 -> delay_a0/1
  bias_a/1 -> downsample_a15/1, downsample_a14/1, downsample_a13/1, downsample_a12/1, downsample_a11/1, downsample_a10/1, downsample_a9/1, downsample_a8/1, downsample_a7/1, downsample_a6/1, downsample_a5/1, downsample_a4/1, downsample_a3/1, downsample_a2/1, downsample_a1/1, downsample_a0/1
  gain_a/1 -> bias_a/1
  sim_a/1 -> gain_a/1

== system xps_library/ADCs/conv ==
  In1 : Inport
  Concat : xbsIndex_r4/Concat  num_inputs=2  dbl_ovrd=off  block_type=concat
      settings: block_version=8.2.02
  Inverter : xbsIndex_r4/Inverter  en=off  latency=0  dbl_ovrd=off  block_type=inv
      settings: xl_area=[0, 0, 0, 0, 0, 0, 0]  block_version=8.2.02
  Reinterpret : xbsIndex_r4/Reinterpret  force_arith_type=on  arith_type="Signed  (2's comp)"  force_bin_pt=on  bin_pt=bit_width-1  block_type=reinterpret
      settings: infoedit="Changes signal type without altering the binary representation.   You can changed the signal between signed and unsigned, and relocate the binary point.<br><br>Hardware notes: In hardware this block costs nothing.<br><br>Example:  Suppose the input is 6 bits wide, signed, with 2 fractional bits, and the output is forced to unsigned with 0 fractional bits.  Then an input of -2.0 (1110.00 in binary 2's complement) becomes an output of 56 (111000 in binary)."  block_version=8.2.02
  Slice : xbsIndex_r4/Slice  nbits=1  boolean_output=off  mode=Upper Bit Location + Width  bit1=0  base1=MSB of Input  bit0=0  base0=LSB of Input  dbl_ovrd=off  block_type=slice
      settings: infoedit="Extracts a given range of bits from each input sample and presents it at the output.  The output type is ordinarily unsigned with binary point at zero, but can be Boolean when the slice is one bit wide.<P><P>Hardware notes: In hardware this block costs nothing."  block_version=8.2.02
  Slice1 : xbsIndex_r4/Slice  nbits=bit_width-1  boolean_output=off  mode=Lower Bit Location + Width  bit1=0  base1=MSB of Input  bit0=0  base0=LSB of Input  dbl_ovrd=off  block_type=slice
      settings: block_version=8.2.02
  Out1 : Outport
  wires:
  Reinterpret/1 -> Out1/1
  Concat/1 -> Reinterpret/1
  Slice1/1 -> Concat/2
  Inverter/1 -> Concat/1
  Slice/1 -> Inverter/1
  In1/1 -> Slice/1, Slice1/1

== system xps_library/ADCs/of1 ==
  s0 : Inport
  s1 : Inport  Port=2
  Compare To Constant1 : simulink/Logic and Bit Operations/Compare To Constant  SystemSampleTime=-1  relop=>  const=2^n_adc_bits-1  LogicOutDataTypeMode=boolean  ZeroCross=off
  Compare To Constant2 : simulink/Logic and Bit Operations/Compare To Constant  SystemSampleTime=-1  relop=>  const=2^n_adc_bits-1  LogicOutDataTypeMode=boolean  ZeroCross=off
  Compare To Constant6 : simulink/Logic and Bit Operations/Compare To Constant  SystemSampleTime=-1  relop=<  const=0  LogicOutDataTypeMode=boolean  ZeroCross=off
  Compare To Constant7 : simulink/Logic and Bit Operations/Compare To Constant  SystemSampleTime=-1  relop=<  const=0  LogicOutDataTypeMode=boolean  ZeroCross=off
  Gain : Gain  Gain=2^(bit_num)
  Logical Operator1 : Logic  Operator=OR  Inputs=4  AllPortsSameDT=off  OutDataTypeStr=boolean
  of : Outport
  wires:
  Gain/1 -> of/1
  s1/1 -> Compare To Constant2/1, Compare To Constant7/1
  Logical Operator1/1 -> Gain/1
  s0/1 -> Compare To Constant1/1, Compare To Constant6/1
  Compare To Constant6/1 -> Logical Operator1/1
  Compare To Constant1/1 -> Logical Operator1/2
  Compare To Constant7/1 -> Logical Operator1/3
  Compare To Constant2/1 -> Logical Operator1/4

== system xps_library/ADCs/of_detect_bus ==
  s0 : Inport
  s1 : Inport  Port=2
  s2 : Inport  Port=3
  s3 : Inport  Port=4
  s4 : Inport  Port=5
  s5 : Inport  Port=6
  s6 : Inport  Port=7
  s7 : Inport  Port=8
  Add : Sum  Inputs=++++
  of1 : casper_library_misc/of1  SystemSampleTime=-1  bit_num=0  n_adc_bits=8
  of2 : casper_library_misc/of1  SystemSampleTime=-1  bit_num=0  n_adc_bits=8
  of3 : casper_library_misc/of1  SystemSampleTime=-1  bit_num=0  n_adc_bits=8
  overflow : Outport
